simulink model "ALGO_Tanker_new_5Pin_baseline"  (R2023a)
settings: Solver=VariableStepAuto  StartTime=0  StopTime=60  RelTol=1e-3
StopFcn:
  | CompareSimResult_baseline
libraries: simulink x18, Solver_SF x1
(part 2 of 2)

== matlab function ALGO_Tanker_new_5Pin_baseline/5DOF牵引车半挂车模型 50%液体 单摆模拟/SP_Model_50per ==
  data: ddy input; ExForce output; ddF input; Theta output
function [ExForce,Theta] = SP_Model(ddy,ddF)
persistent sim_param Ts y0
%% 定义摆
if isempty(Ts)
%SP模型，共5个参数拟合
% 参数 m1 h0 hp lp coeff
x=[10890,1.5,0.13,0.97,0.13];
% 获取参数
sim_param=getParam_SP(x);
%初始状态量
y0=zeros(9,1);
%采样时间
Ts=0.005;
end

y=y0;

%% 求解微分方程
dy=zeros(9,1);
dy(1)=y(2);
dy(2)=ddy;
dy(3)=(dy(2)-y(3))/Ts;
dy(4)=y(5);
dy(5)=ddF;
dy(6)=(dy(5)-y(6))/Ts;
dy(7)=y(8);
dy(8)=calc_ddth_SP(y,sim_param);
dy(9)=(dy(8)-y(9))/Ts;
y=y0+dy*Ts;
%% 计算三向力输出
[Fy,Fz,Mx]=calc_Fp_SP(y,sim_param);
ExForce=[Fy,Fz,Mx];
%% 更新状态量
y0=y;
th=y(7);
dth=y(8);
Theta=[th,dth];
end

%% 根据变量获取参数
function sim_param=getParam_SP(x)
%根据变量生成传输参数
TotMass=14462;
m1=x(1);%参数1
m0=TotMass-m1;
h0=x(2);%参数2
hp=x(3);%参数3
lp=x(4);%参数4
g=9.806;
coeff=x(5);%参数5
sim_param=[m0,m1,h0,hp,lp,g,coeff];
end

%% 求解三向力输出
function [Fy,Fz,Mx] = calc_Fp_SP(state,param)
% sim_param=[m0,m1,h0,hp,lp,g,coeff];
m0=param(1);
m1=param(2);
h0=param(3);
hp=param(4);
lp=param(5);
g=param(6);
% co=param(7);

% y=state(1);
% dy=state(2);
ddy=state(3);
f=state(4);
df=state(5);
ddf=state(6);
th=state(7);
dth=state(8);
ddth=state(9);

%定义运算符简写
sf=sin(f);
cf=cos(f);
s2=sin(th+f);
c2=cos(th+f);
L=lp+hp;
%定义质量块的 位置矢量
exh=0.77; %额外增加的高度是罐底到力矩受力中心车轴中心的高度
R0=[-(h0+exh)*sf,(exh+h0)*cf];

R1=[-(L+exh)*sf+lp*s2
    (L+exh)*cf-lp*c2];

ddRp0=[ddy-h0*cf*ddf+df^2*h0*sf
-h0*sf*ddf-h0*cf*df^2+g];

ddRp1=[ddy+ddf*(-L*cf+lp*c2)+ddth*(lp*c2)+df^2*(L*sf-lp*s2)+dth^2*(-lp*s2)+df*dth*(-2*lp*s2)
ddf*(-L*sf+lp*s2)+ddth*(lp*s2)+df^2*(-L*cf+lp*c2)+dth^2*(lp*c2)+df*dth*(2*lp*c2)+g];

Fp=m0*ddRp0+m1*ddRp1;
Fy=Fp(1)*cf-(-Fp(2))*sf;
Fz=(-Fp(2))*cf+Fp(1)*sf;
Mx0=(m0*(R0(1)*-ddRp0(2)+R0(2)*ddRp0(1)));
Mx1=(m1*(R1(1)*-ddRp1(2)+R1(2)*ddRp1(1)));

Mx=Mx0+Mx1;

end
%% 求解ddth
function ddth = calc_ddth_SP(state,param)
% sim_param=[m0,m1,h0,hp,lp,g,coeff];
% m0=param(1);
% m1=param(2);
% h0=param(3);
hp=param(4);
lp=param(5);
g=param(6);
co=param(7);

% y=state(1);
% dy=state(2);
ddy=state(3);
f=state(4);
df=state(5);
ddf=state(6);
th=state(7);
dth=state(8);
% ddth=state(9);


%定义运算符简写
s1=sin(th);
c1=cos(th);
s2=sin(th+f);
c2=cos(th+f);
L=lp+hp;

ddth=-(ddy*lp*c2+ddf*(-lp*L*c1+lp^2)-df^2*lp*L*s1+g*lp*s2)/(lp^2);
ddth=ddth-co*dth;

end

== matlab function ALGO_Tanker_new_5Pin_baseline/5DOF牵引车半挂车模型 50%液体 单摆模拟/TrailorTruck_5DOF_SP_50per ==
  data: vx input; state output; delta input; observe output
function [state,observe]=TrailorTruck_5DOF_SP(vx,delta)
%% 初始状态定义
%要记得设置本模块的采样时间哦
persistent Ts                             %采样时间    
persistent state0                         %上一时刻状态
if isempty(state0)
   Ts=0.01;%采样时间
   %初始化状态量
   vx10=vx(1);vx20=vx(2);
   vy10=0; df10=0;F10=0;dF10=0; Y10=0;X10=0;f10=0; %牵引车状态变量
   vy20=0; df20=0;F20=0;dF20=0; Y20=0;X20=-5.638315;f20=0;%半挂车状态变量
   th0=0; dth0=0;%等效摆状态变量
   state0=[vy10,df10,F10,dF10,vy20,df20,F20,dF20,...
       th0,dth0,f10,f20,vx10,vx20,Y10,X10,Y20,X20]';
   
end
%% 定义动力学模型参数
persistent a b c d e                    %轴距纵向几何参数
persistent Tw1 Tw2                      %轮距横向几何参数
persistent h1 h2 hc1 hc2                %质心至侧倾轴线距离
                                        %铰接点至侧倾轴线距离
persistent m1 m2 m1s m2s g;g=9.806;
persistent I1zz I1xx I1xz I2zz I2xx I2xz %惯性参量
persistent k1 k2 k3                      %线性轮胎模型参数
persistent kr1 kr2 c1 c2 k12             %悬架模型参数
persistent m0 mp h0 hp lp co             %等效摆模型参数
if isempty(a)
%摆模型参数
x=[10890,1.5,0.13,0.97,0.13];
sim_param=getParam_SP(x);
% sim_param=[m0,m1,h0+0.77,hp+0.77,lp,g,coeff];
m0=sim_param(1);
mp=sim_param(2);
h0=sim_param(3);
hp=sim_param(4);
lp=sim_param(5);
co=sim_param(7);
%车辆模型参数
L1=(5+6.27)/2;L2=(10.15+11.5)/2;       %轴距平均
a=1.385;b=L1-a;c=5.635-a;e=5.5;d=L2-e; %纵向几何
Tw1=(2.03+1.863*2)/3;Tw2=1.863;        %轮距平均
hm1s=1.02; %牵引车质心高度
hm2s=1.58; %50%充液率时半挂车质心高度
hhitch=1.1;%交接点高度
hroll1=0.2314;hroll2=0.9630;           %侧倾中心高度
h1=hm1s-hroll1;h2=hm2s-hroll2;hc1=hhitch-hroll1;hc2=hhitch-hroll2;%高度几何
m1s=6310;m1=m1s+570+785*2;             %牵引车质量
% m2s=5925;m2=m2s+665*2;               %半挂车空载质量
m2s=20387;m2=m2s+665*2;
I1xx=6879;I1xz=130;I1zz=19665;         %牵引车惯量
% I2xx=9960;I2xz=0;I2zz=179992;        %半挂车惯量
I2xx=9960;I2xz=0;I2zz=331380;
%轮胎模型参数
k1=-37e4;k2=-82e4;k3=-80e4;             %侧偏刚度
kr1=18.7e5;kr2=9.14e5;k12=68.3e5;       %侧倾刚度
c1=64.4e3;c2=197.7e3;                   %悬架等效阻尼
end
%% 定义线性动力学模型
dF2=state0(8);f1=state0(11);f2=state0(12);
vx1=vx(1);vx2=vx(2);
%线性车辆动力学模型
% M*dX = A0*X + B0*u
m14=-m1s*h1*c-I1xz;
m21=m1*vx1*hc1-m1s*h1*vx1;
m24=I1xx+2*m1s*h1^2-m1s*h1*hc1;
m55=m2*vx2*hc2-m2s*h2*vx2;
m58=I2xx+2*m2s*h2^2-m2s*h2*hc2;

M=[m1*vx1*c, I1zz, 0,   m14,     0,        0,   0,     0;
    m21,    -I1xz, 0,   m24,     0,        0,   0,     0;
   m1*vx1,      0, 0, -m1s*h1, m2*vx2,     0,   0, -m2s*h2;
     0,         0, 0,     0,  m2*vx2*e, -I2zz,  0, I2xz-m2s*h2*e;
     0,         0, 0,     0,    m55,    -I2xz,  0,    m58;
     1,    -c/vx1, 0, -hc1/vx1,  -1,   -e/vx2,  0, hc2/vx2;
     0,         0, 1,     0,     0,        0,   0,     0;
     0,         0, 0,     0,     0,        0,   1,     0   ];
 
 a11 = (c+a)*k1 + (c-b)*k2;
 a12 = a*(c+a)*k1/vx1 - b*(c-b)*k2/vx1 - m1*vx1*c;
 a22 = (a*k1-b*k2)*hc1/vx1 + (m1s*h1-m1*hc1)*vx1;
 a23 = m1s*g*h1 - kr1 -k12;
 a32 = (a*k1-b*k2)/vx1 - m1*vx1;
 a36 = -d*k3/vx2 - m2*vx2;
 a46 = -d*(e+d)*k3/vx2 - m2*vx2*e;
 a56 = (m2s*h2-m2*hc2)*vx2 - d*k3*hc2/vx2;
 a57 = m2s*g*h2 - kr2 -k12;
 %  X=   b1     df1    F1  dF1        b2  df2, F2   dF2 
 Acm0=[ a11,    a12,    0,   0,       0,   0,  0,    0;
   (k1+k2)*hc1, a22,  a23, -c1,       0,   0, k12,   0;
     k1+k2,     a32,    0,   0,      k3,  a36, 0,    0;
        0,       0,     0,   0, (e+d)*k3, a46, 0,    0;
        0,       0,    k12,  0,   k3*hc2, a56, a57, -c2;
        0,      -1,     0,   0,       0,   1,  0,    0;
        0,       0,     0,   1,       0,   0,  0,    0;
        0,       0,     0,   0,       0,   0,  0,    1   ];
    
 Bcm0=[-(c+a)*k1, -k1*hc1, -k1, 0, 0, 0, 0, 0]';
 

 %       1    2   3    4    5    6    7    8   9  10
%  X = vy1,  df1,F1, dF1, vy2, df2,  F2, dF2, th dth
% dX = dvy1;ddf1;dF1;ddF1;dvy2;ddf2;dF2;ddF2;dth;ddth ←M_
M_=zeros(10);
M_(9,9)=1;
M_(10,:)=[0,0,0,0,vx2/lp,0,0,hp/lp,0,1];
M_(3,:)=[0,0,0,0,(mp+m0)*vx2,0,(m0*h0+mp*(hp+lp))*dF2^2,-(m0+h0+mp*hp),0,mp*lp];
M_(4,:)=M_(3,:)*e;
M_(5,:)=M_(3,:)*hc2+...
[0,0,0,0,-(m0*h0+mp*hp)*vx2,0,0,(m0+h0^2+mp*hp^2),0,-mp*lp*hp];

A_=zeros(10);
A_(9,10)=1;
A_(10,:)=[0,0,0,0,0,-vx2/lp,0,0,-(hp/lp+1)*dF2^2-g/lp,-co];
A_(3,:)=[0,0,0,0,0,-(mp+m0)*vx2,0,0,0,0];
A_(4,:)=A_(3,:)*e;
A_(5,:)=A_(3,:)*hc2+...
[0,0,0,0,0,(m0*h0+mp*hp)*vx2,0,0,-mp*lp*g,0];
%       1    2   3    4    5    6    7    8   9  10
%  X =  0,   0,  0,   0,   0, df2,   0,   0, th  0
% dX =  0;   0;  0;   0;dvy2;   0;dF2;ddF2;dth;  0
 Acm=([M,zeros(8,2);zeros(2,10)]+M_)\([Acm0,zeros(8,2);zeros(2,10)]+A_);
 Bcm=([M,zeros(8,2);zeros(2,10)]+M_)\[Bcm0;zeros(2,1)];
 
 %% 增广状态量 并转变bi为vyi
 
 Trans=diag([vx1,1,1,1,vx2,1,1,1,1,1]);
 Ac=[Trans*Acm,zeros(10,8);            %增广状态量后的矩阵
     0,1,0,0,0,0,0,0,0,0,0,0,0,0,0,0,0,0;
     0,0,0,0,0,1,0,0,0,0,0,0,0,0,0,0,0,0;
     zeros(2,18);
     cos(f1),0,0,0,0,0,0,0,0,0,0,0,sin(f1),0,0,0,0,0;
    -sin(f1),0,0,0,0,0,0,0,0,0,0,0,cos(f1),0,0,0,0,0;
     0,0,0,0,cos(f2),0,0,0,0,0,0,0,0,sin(f2),0,0,0,0;
    0,0,0,0,-sin(f2),0,0,0,0,0,0,0,0,cos(f2),0,0,0,0  ];

 Bc=[Trans*Bcm;zeros(8,1)] ;
 
 %% 离散化线性模型
 [A,B]=c2d_zoh(Ac,Bc,Ts);             %离散化线性模型
 
%       1   2    3    4   5    6    7    8    9  10   11  12  13  14 15 16
% dX=[dvy1;ddf1;dF1;ddF1;dvy2;ddf2;dF2;ddF2;df1;df2;dvx1;dvx2;dY1;dX2;dY2;dX2];
%维度：14×1 

%% 更新状态量
%组装状态量
state=A*state0+B*delta;  %进行下一步更新
%% 观测量计算
%观测量为 Y1 X1 f1 th dth LTR1 LTR2
obsvMat=[zeros(2,14),eye(2),zeros(2,2); % Y1 X1
         zeros(1,10),1,zeros(1,7);      % f1
         zeros(2,8),eye(2),zeros(2,8);  % th dth
         2/(Tw1*m1*g)*[0,0,-(kr1+k12),-c1,0,0,k12,0],zeros(1,10);%LTR1
         2/(Tw2*m2*g)*[0,0,k12,0,0,0,-(kr2+k12),-c2],zeros(1,10);%LTR2
         ];
observe=obsvMat*state;
%% 拆解状态量并为下一步计算保存

state0=state;



end
%% 根据变量获取参数
function sim_param=getParam_SP(x)
%根据变量生成传输参数
TotMass=14462;
m1=x(1);%参数1
m0=TotMass-m1;
h0=x(2);%参数2
hp=x(3);%参数3
lp=x(4);%参数4
g=9.806;
coeff=x(5);%参数5
sim_param=[m0,m1,h0+0.77,hp+0.77,lp,g,coeff];
end

== matlab function ALGO_Tanker_new_5Pin_baseline/LTR_calc  ==
  data: TireFz input; LTR output
function LTR = fcn(TireFz)
% 分配物理量
FzL=sum(TireFz(1:5));
FzR=sum(TireFz(6:10));
% 进行计算
LTR=(FzL-FzR)/(FzL+FzR);
end
